simulink model "Sample"  (R2021b)
settings: Solver=VariableStepAuto  StartTime=0.0  StopTime=10.0  RelTol=1e-3
settings Model: Creator=ygkwon  LastModifiedBy=ygkwon

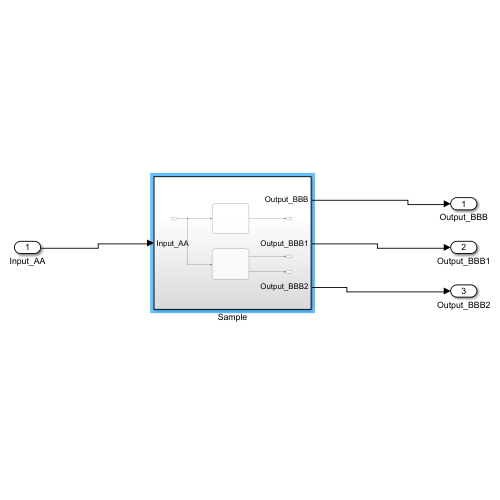
[thumbnail: Simulink's stored preview of the top-level diagram]
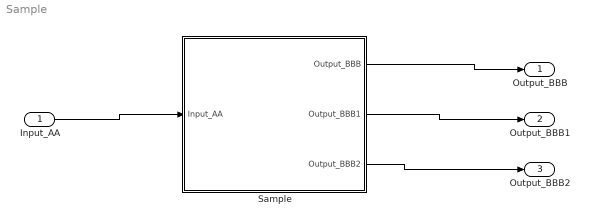
== system Sample ==
  Input_AA : Inport
  Sample : Subsystem
  Output_BBB : Outport
  Output_BBB1 : Outport  Port=2
  Output_BBB2 : Outport  Port=3
  wires:
  Input_AA/1 -> Sample/1(Input_AA)
  Sample/1(Output_BBB) -> Output_BBB/1
  Sample/2(Output_BBB1) -> Output_BBB1/1
  Sample/3(Output_BBB2) -> Output_BBB2/1

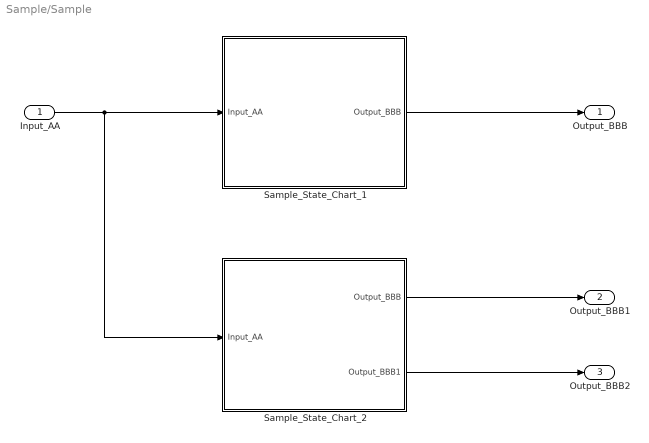
== system Sample/Sample ==
  Input_AA : Inport
  Sample_State_Chart_1 : Stateflow chart  TreatAsAtomicUnit=on
  Sample_State_Chart_2 : Stateflow chart  TreatAsAtomicUnit=on
  Output_BBB : Outport
  Output_BBB1 : Outport  Port=2
  Output_BBB2 : Outport  Port=3
  wires:
  Input_AA/1 -> Sample_State_Chart_2/1(Input_AA), Sample_State_Chart_1/1(Input_AA)
  Sample_State_Chart_1/1(Output_BBB) -> Output_BBB/1
  Sample_State_Chart_2/1(Output_BBB) -> Output_BBB1/1
  Sample_State_Chart_2/2(Output_BBB1) -> Output_BBB2/1

== stateflow chart Sample/Sample_State_Chart_1 ==
  state Sample_State_Chart_2222
    en:
    Output_BBB = 22;
    state a
      en:
      Output_BBB=1;
    state a1
      en:
      Output_BBB=2;
    state a2
      en:
      Output_BBB=1;
    state a3
      en:
      Output_BBB=2;
      du:
      hello();
    (default) -> a [order 1] : [Input_AA == 11]
    a1 -> a [order 1] : [Input_AA==1]
    a1 -> a [order 2] : [Input_AA==11]
    a -> a1 : [Input_AA==2]
    (default) -> a2 [order 2]
    a3 -> a2 [order 1] : [Input_AA==1]
        | %hello
    a3 -> a2 [order 2] : [Input_AA==11]
    a2 -> a3 : [Input_AA==2]
  state hello [function]
    (default) -> (junction 20)
    (junction 20) -> (junction 24) [order 1] : [Input_AA == 111]
    (junction 20) -> (junction 22) [order 2]
    (junction 24) -> (junction 26) : {Output_BBB = 333;}
    (junction 26) -> (junction 22)
    (junction 22) -> (junction 29)
  data: Input_AA input; Output_BBB output

== stateflow chart Sample/Sample_State_Chart_2 ==
  state Sample_State_Chart_3
    state b2
      en:
      Output_BBB1=1;
    state b3
      en:
      Output_BBB1=2;
    state a4
      en:
      Output_BBB1=1;
    state a5
      en:
      Output_BBB1=2;
    (default) -> b2 [order 1] : [Input_AA == 11]
    b3 -> b2 [order 1] : [Input_AA==1]
    b3 -> b2 [order 2] : [Input_AA==11]
    b2 -> b3 : [Input_AA==2]
    (default) -> a4 [order 2]
    a5 -> a4 [order 1] : [Input_AA==1]
        | %hello
    a5 -> a4 [order 2] : [Input_AA==11]
    a4 -> a5 : [Input_AA==2]
  data: Input_AA input; Output_BBB output; Output_BBB1 output double
